simulink model "cstr_sim"  (R2017a)
settings: Solver=ode45  StartTime=0.0  StopTime=10  RelTol=1e-3  EnableMultiTasking=on
StopFcn:
  | plot_reactor
libraries: simulink x5
settings Model: Creator=tsladeche  LastModifiedBy=ljxia_000
settings DataIOCC: LimitDataPoints=on  SaveFormat=Array  SignalLoggingSaveFormat=ModelDataLogs
settings OptimizationCC: ExpressionDepthLimit=2147483647  LifeSpan=inf
settings DebuggingCC: UnderspecifiedInitializationDetection=Classic  MergeDetectMultiDrivingBlocksExec=none  SolverPrmCheckMsg=warning  FcnCallInpInsideContextMsg=warning  StateNameClashWarn=warning  SFUnexpectedBacktrackingDiag=warning  SFNoUnconditionalDefaultTransitionDiag=warning  SFExecutionAtInitializationDiag=none
settings HardwareCC: ProdBitPerPointer=32  ProdBitPerSizeT=32  ProdBitPerPtrDiffT=32  ProdLargestAtomicFloat=None  ProdIntDivRoundTo=Undefined  ProdEndianess=Unspecified  ProdWordSize=32  ProdHWDeviceType=32-bit Generic
settings ModelReferenceCC: PropagateSignalLabelsOutOfModel=off
settings GRTTargetCC: TargetLangStandard=C89/C90 (ANSI)  GeneratePreprocessorConditionals=Disable all  CombineOutputUpdateFcns=off  GRTInterface=on
settings ConfigComp: CovMetricSettings=dw  CovHtmlReporting=on  CovSaveCumulativeToWorkspaceVar=on  CovSaveSingleToWorkspaceVar=on  CovExternalEMLEnable=off

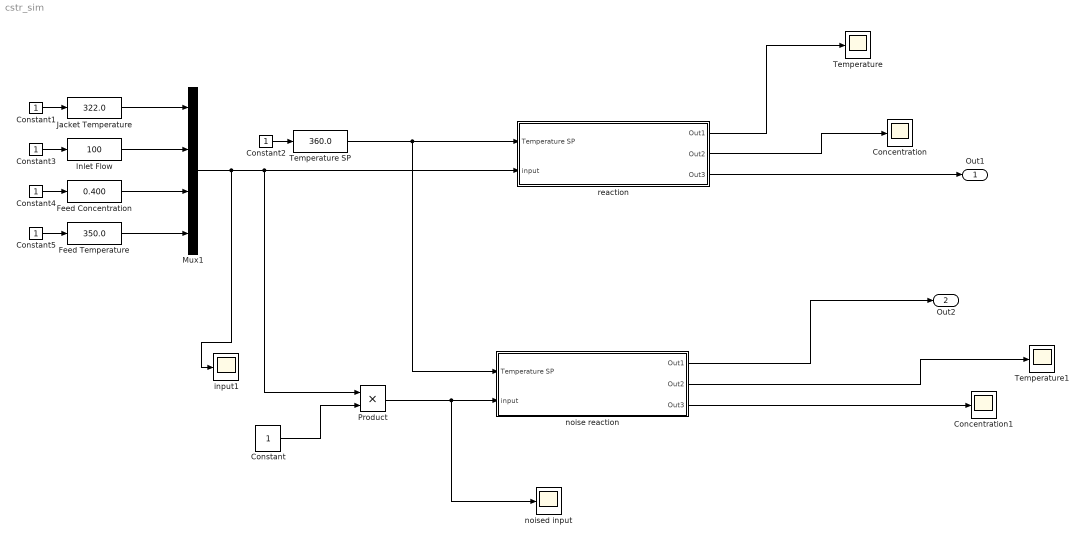
== system cstr_sim ==
  Concentration : Scope
  Concentration1 : Scope
  Constant{,1..5} (6 alike) : Constant  SampleTime=0.01
  Feed Concentration : simulink/Math Operations/Slider Gain  gain=0.400  low=0  high=1
  Feed Temperature : simulink/Math Operations/Slider Gain  gain=350.0  low=300  high=400
  Inlet Flow : simulink/Math Operations/Slider Gain  gain=100  low=0  high=200
  Jacket Temperature : simulink/Math Operations/Slider Gain  gain=322.0  low=250  high=350
  Mux1 : Mux
  Product : Product
  Temperature : Scope
  Temperature SP : simulink/Math Operations/Slider Gain  gain=360.0  low=300  high=400
  Temperature1 : Scope
  input1 : Scope
  noise reaction : Subsystem
  noised input : Scope
  reaction : Subsystem
  Out1 : Outport
  Out2 : Outport  Port=2
  wires:
  Constant3/1 -> Inlet Flow/1
  Constant1/1 -> Jacket Temperature/1
  Inlet Flow/1 -> Mux1/2
  Jacket Temperature/1 -> Mux1/1
  Constant4/1 -> Feed Concentration/1
  Feed Concentration/1 -> Mux1/3
  Constant5/1 -> Feed Temperature/1
  Feed Temperature/1 -> Mux1/4
  Constant2/1 -> Temperature SP/1
  reaction/1(Out1) -> Temperature/1
  reaction/2(Out2) -> Concentration/1
  reaction/3(Out3) -> Out1/1
  Temperature SP/1 -> noise reaction/1(Temperature SP), reaction/1(Temperature SP)
  Mux1/1 -> input1/1, Product/1, reaction/2(input)
  noise reaction/1(Out1) -> Out2/1
  noise reaction/2(Out2) -> Temperature1/1
  noise reaction/3(Out3) -> Concentration1/1
  Product/1 -> noised input/1, noise reaction/2(input)
  Constant/1 -> Product/2

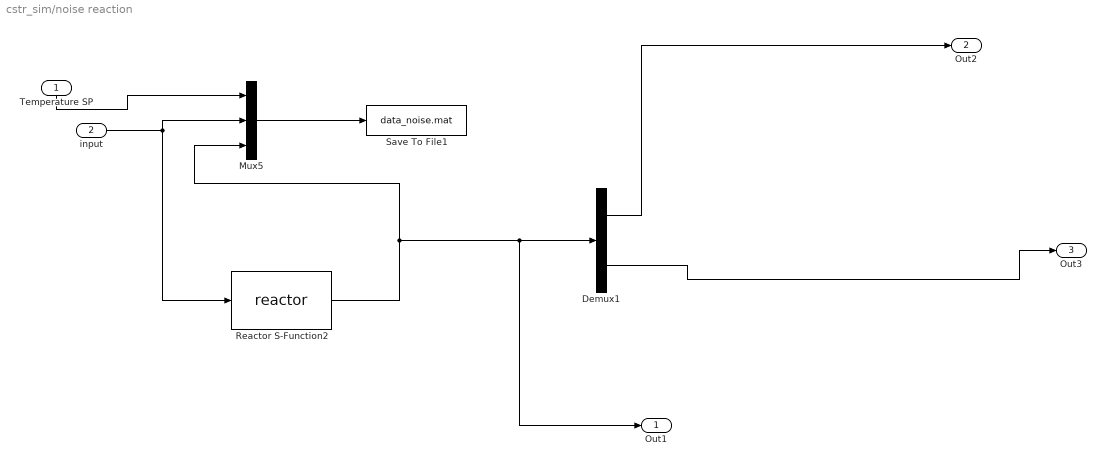
== system cstr_sim/noise reaction ==
  Temperature SP : Inport
  input : Inport  Port=2
  Demux1 : Demux  Outputs=2
  Mux5 : Mux  Inputs=3
  Reactor S-Function2 : S-Function  FunctionName=reactor  SFunctionDeploymentMode=off  EnableBusSupport=off
  Save To File1 : ToFile  Filename=data_noise.mat  MatrixName=cstr  SampleTime=0.01
  Out1 : Outport
  Out2 : Outport  Port=2
  Out3 : Outport  Port=3
  wires:
  Temperature SP/1 -> Mux5/1
  Demux1/2 -> Out3/1
  Reactor S-Function2/1 -> Mux5/3, Out1/1, Demux1/1
  Mux5/1 -> Save To File1/1
  Demux1/1 -> Out2/1
  input/1 -> Mux5/2, Reactor S-Function2/1

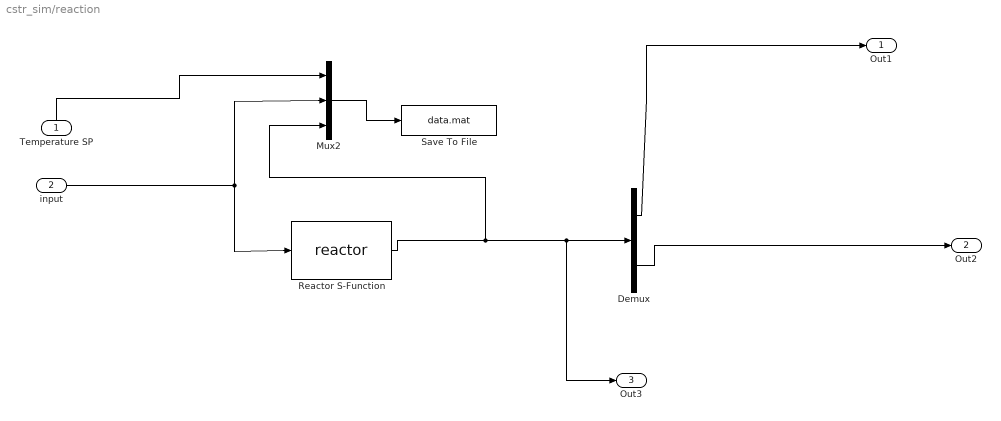
== system cstr_sim/reaction ==
  Temperature SP : Inport
  input : Inport  Port=2
  Demux : Demux  Outputs=2
  Mux2 : Mux  Inputs=3
  Reactor S-Function : S-Function  FunctionName=reactor  SFunctionDeploymentMode=off  EnableBusSupport=off
  Save To File : ToFile  Filename=data.mat  MatrixName=cstr  SampleTime=0.01
  Out1 : Outport
  Out2 : Outport  Port=2
  Out3 : Outport  Port=3
  wires:
  Reactor S-Function/1 -> Mux2/3, Out3/1, Demux/1
  Demux/2 -> Out2/1
  Demux/1 -> Out1/1
  Mux2/1 -> Save To File/1
  input/1 -> Reactor S-Function/1, Mux2/2
  Temperature SP/1 -> Mux2/1
